simulink model "ARS308_RX"  (R2018b)
settings: Solver=FixedStepAuto  StartTime=0.0  StopTime=inf  FixedStep=0.005  RelTol=1e-3
PostLoadFcn:
  | if any(exist('dsrtsu_mdlpostloadfcn', 'file') ~= 0), dsrtsu_mdlpostloadfcn('Execute', bdroot); end
libraries: rtican x18
(part 3 of 4)

== system ARS308_RX/Subsystem/Function-Call Subsystem3 ==
  function : TriggerPort  TriggerType=function-call  VariantControl=Variant
  Cast To Single : DataTypeConversion  OutDataTypeStr=single
  Cast To Single1 : DataTypeConversion  OutDataTypeStr=single
  Cast To Single2 : DataTypeConversion  OutDataTypeStr=single
  Obj_0_Status : rtican/RTICAN Receive (RX)   Reserved1=[]  Reserved2=[]  Reserved3=[]  Reserved4=[]  SfcnMessage=[]  Msg_Struct=[]  BoardTypeNo=[]  BoardNo=[]  ChannelNo=[]  Parameters=[]  DialogFcn=[]  UnitName=[]  Revision=[]  UnitValues=[]  DSProperties=struct('RTI',struct('Version',uint32(5),'BlockType',struct('isSLSource',uint8(1),'isSLSink',uint8(1),'isHWSource',uint8(0),'isHWSink',uint8(0),'isSetup',uint8(0),'isInline',uint8(1),'isNonInline',uint8(0),'isInterrupt',uint8(0),'isChannelwise',uint8(0)),'IOBoardType','RTICAN','UnitType','MESSAGE','Identifier','RX','DialogType','MSVC','BlockSet','RTICAN','SlaveProcessor','CAN'))  RTIBlockInterface=struct('OutputPortsWidth',int32([1 1 1 1 1 1]),'OutputPortsActive',[1 1 1 1 1 1],'OutputPortsName',{{'Obj_InterfaceVersion','Obj_MeasCounter','Obj_NofObjects',['RX status'],['RX time'],['RX delta time']}},'OutputPortsDataType',{{'SS_DOUBLE','SS_DOUBLE','SS_DOUBLE','SS_DOUBLE','SS_DOUBLE','SS_DOUBLE'}},'OutputPortsLabel',{{'Obj_InterfaceVersion','Obj_MeasCounter','Obj_NofObjects','','',''}},'OutputPortsLabelMode','ON','InputPortsWidth',int32(0),'InputPortsActive',0,'DialogFcn','rtican_message_interface_gui','BlockDisplay',{{'','center'}},'IconTransparency','on','ParameterTunableNames',{{}},'InitLevel',3,'BlockName',struct('Token',{{'Obj_0_Status'}}),'SampleTime',{{-1}},'TriggerPort',{{'none'}},'EnablePort',{{'none'}})  RTIBlockParameters=struct('BoardTypeNo',{{1,'OFF',[]}},'BoardNo',{{3,'ON',[1 16]}},'ChannelNo',{{2,'ON',[1 2]}},'Parameters',{{struct('DataFileSupport',struct('DataFileSelectedMaster',1,'DataFileSelectedLocal',1,'DataFileName',['c:\users\石丽\desktop\zone\2020_demo\308\ars408_can_database_ch2 -new.dbc|c:\users\石丽\desktop\zone\2020_demo\308\ars408_can_database_ch0 -new.dbc|c:\users\石丽\desktop\zone\2020_demo\308\ars408_can_database_ch1-new.dbc|c:\users\石丽\desktop\zone\2020_demo\308\ars408_can_database_ch3-new.dbc|'],'DataFileDate',{{{['18-12月-2020 14:05:28']},{['18-12月-2020 14:05:27']},{['18-12月-2020 14:05:27']},{['18-12月-2020 14:05:26']}}},'SelectedFile','c:\users\石丽\desktop\zone\2020_demo\308\ars408_can_database_ch3-new.dbc'),'Options',struct('StatusSelected',1,'TimeSelected',1,'DeltaTimeSelected',1,'BytePortSelected',0,'MessageLengthSelected',0,'TriggerPort',struct('Selected',0,'TriggerType',0),'UserCoding',struct('Selected',0,'InterfaceFile','UserDecodingFile','FcnName','UserDecodeFcn','InportSelected',0,'InportWidth',1,'OutportSelected',0,'OutportWidth',1),'EnablePortSelected',0,'SignalOnPortnameSelected',1,'UseRXService',0),'Message',struct('MsgOnBlocknameSelected',1,'MsgName','Obj_0_Status','MsgIdFormat',0,'MsgId',1594,'MsgLength',4,'NumSignals',3,'SampleTime',-1,'Signal',struct('SgnName',{'Obj_InterfaceVersion','Obj_MeasCounter','Obj_NofObjects'},'SgnStartBit',{4,8,24},'SgnLength',{4,16,8},'SgnType',{0,0,0},'ModeValue',{-1,-1,-1},'DataType',{0,0,0},'ByteLayout',{2,2,2},'Factor',{1,1,1},'Offset',{0,0,0},'SgnComment',{{['Object CAN Interface Version Number']},{['Measurement Counter']},{['Number of Objects sent']}},'SgnUnit',{'','',''},'Min',{0,0,0},'Max',{16,65535,255},'SLDataType',{'SS_DOUBLE','SS_DOUBLE','SS_DOUBLE'}),'MsgIdNumFormat',1,'MsgComment',{{['Status information about object']}}),'Version',1.2,'general',struct('isFromLib',0)),'OFF',[]}},'GroupId',{{struct('Group',{{'RTICAN'}},'No',1,'Behavior',{{'NAMECHANGE'}},'BlockType',{{'SINK'}},'NameChangeFlag',0),'OFF',[]}},'SFcnRTICANMessage',{{struct('MsgType','RX','SFcnPortType','Scalar','MsgName','Obj_0_Status','MsgIdFormat','STD','MsgId',1594,'MsgLength',4,'NumSignals',3,'SampleTime',-1,'Signal',struct('SgnName',{'Obj_InterfaceVersion','Obj_MeasCounter','Obj_NofObjects'},'SgnStartBit',{4,8,24},'SgnLength',{4,16,8},'SgnType',{'standard','standard','standard'},'ModeValue',{-1,-1,-1},'DataType',{['unsigned int'],['unsigned int'],['unsigned int']},'ByteLayout',{['motorola back.'],['motorola back.'],['motorola back.']},'Factor',{1,1,1},'Offset',{0,0,0},'SLDataType',{'SS_DOUBLE','SS_DOUBLE','SS_DOUBLE'}),'StatusSelected','yes','TimeSelected','yes','DeltaTimeSelected','yes','BytePortSelected','no','MessageLengthSelected','no','TriggerPort',struct('Selected','no','TriggerType',0),'UserCoding',struct('Selected','no','InterfaceFile','UserDecodingFile','FcnName','UserDecodeFcn','InportSelected','no','InportWidth',1,'OutportSelected','no','OutportWidth',1),'EnablePortSelected','no','UseRXService','no','BoardType','DS1','BoardNo',3,'ControllerNo',2),'OFF',[]}},'TLCFileName',{{'rtican_rx_message','OFF',[]}})  RTISFcnParameters=struct('SFcnRTICANMessage','struct','TLCFileName','char')  RTIBlockParaDefault=struct('BoardTypeNo',4302,'BoardNo',1,'ChannelNo',1,'Parameters',struct('DataFileSupport',struct('DataFileSelectedMaster',0,'DataFileSelectedLocal',0,'DataFileName','','DataFileDate','','SelectedFile',['<no file selected>']),'Options',struct('StatusSelected',1,'TimeSelected',1,'DeltaTimeSelected',1,'BytePortSelected',0,'MessageLengthSelected',0,'TriggerPort',struct('Selected',0,'TriggerType','rising'),'UserCoding',struct('Selected',0,'InterfaceFile','UserDecodingFile','FcnName','UserDecodeFcn','InportSelected',0,'InportWidth',1,'OutportSelected',0,'OutportWidth',1),'EnablePortSelected',0,'SignalOnPortnameSelected',1,'UseRXService',0),'Message',struct('MsgOnBlocknameSelected',0,'MsgName',['RX Message'],'MsgIdFormat',0,'MsgId',100,'MsgLength',8,'NumSignals',1,'SampleTime',-1,'Signal',struct('SgnName',['RX signal'],'SgnStartBit',0,'SgnLength',8,'SgnType',0,'ModeValue',-1,'DataType',0,'SLDataType','SS_DOUBLE','ByteLayout',0,'Factor',1,'Offset',0,'Min',0,'Max',255,'SgnComment',{{}},'SgnUnit',''),'MsgIdNumFormat',0,'MsgComment',{{''}}),'Version',1.2,'general',struct('isFromLib',1)),'GroupId',struct('Group',{{'RTICAN'}},'No',1,'Behavior',{{'NAMECHANGE'}},'BlockType',{{'SINK'}},'NameChangeFlag',0),'SFcnRTICANMessage',struct('MsgType','RX','MsgName',['RX Message'],'MsgIdFormat','STD','MsgId',100,'MsgLength',8,'NumSignals',1,'SampleTime',-1,'Signal',struct('SgnName',['RX signal'],'SgnStartBit',0,'SgnLength',8,'SgnType','standard','ModeValue',-1,'DataType',['unsigned int'],'ByteLayout',['little endian'],'SLDataType','SS_DOUBLE','Factor',1,'Offset',0),'StatusSelected','yes','TimeSelected','yes','DeltaTimeSelected','yes','BytePortSelected','no','MessageLengthSelected','no','EnablePortSelected','no','UserCoding',struct('Selected','no','InterfaceFile','UserDecodingFile','FcnName','UserDecodeFcn','InportSelected','no','InportWidth',1,'OutportSelected','no','OutportWidth',1),'TriggerPort',struct('Selected','no','TriggerType','rising'),'UseRXService','no','BoardType','DS4302','BoardNo',1,'ControllerNo',1,'SFcnPortType','Scalar'),'TLCFileName','rtican_rx_message')
      settings: AttributesFormatString=Group Id: RTICAN1\n  SourceProductName=dSPACE RTI CAN Blockset
  Out1 : Outport
  Out2 : Outport  Port=2
  Out3 : Outport  Port=3
  wires:
  Obj_0_Status/2 -> Cast To Single/1  "Obj_MeasCounter"
  Obj_0_Status/3 -> Cast To Single1/1  "Obj_NofObjects"
  Cast To Single/1 -> Out1/1
  Cast To Single1/1 -> Out2/1
  Obj_0_Status/1 -> Cast To Single2/1  "Obj_InterfaceVersion"
  Cast To Single2/1 -> Out3/1

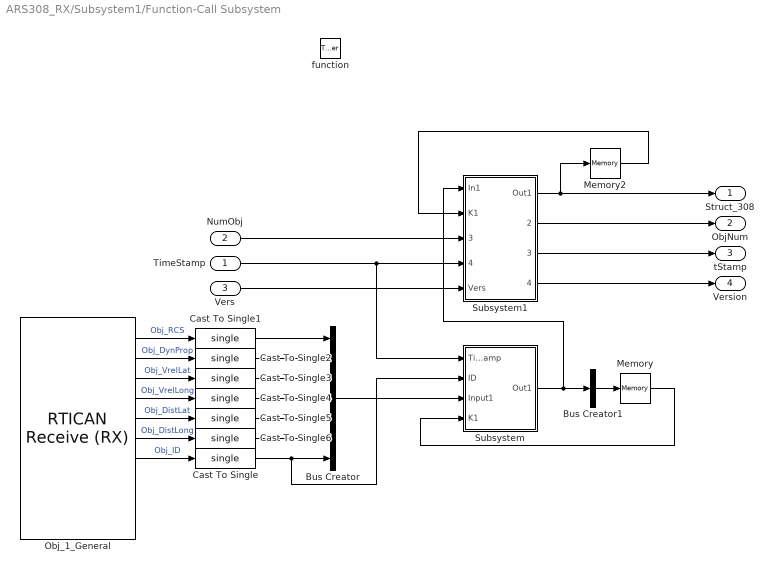
== system ARS308_RX/Subsystem1/Function-Call Subsystem ==
  TimeStamp : Inport
  NumObj : Inport  Port=2
  Vers : Inport  Port=3
  function : TriggerPort  TriggerType=function-call  VariantControl=Variant
  Bus Creator : BusCreator  Inputs=7  OutDataTypeStr=Bus: Bus_308  NonVirtualBus=on
      settings: InheritFromInputs=off
  Bus Creator1 : BusCreator  Inputs=1  OutDataTypeStr=Bus: BusArray_308  NonVirtualBus=on
      settings: InheritFromInputs=off
  Cast To Single{,1..6} (7 alike) : DataTypeConversion  OutDataTypeStr=single
  Memory : Memory  InheritSampleTime=on
  Memory2 : Memory  InheritSampleTime=on
  Obj_1_General : rtican/RTICAN Receive (RX)   Reserved1=[]  Reserved2=[]  Reserved3=[]  Reserved4=[]  SfcnMessage=[]  Msg_Struct=[]  BoardTypeNo=[]  BoardNo=[]  ChannelNo=[]  Parameters=[]  DialogFcn=[]  UnitName=[]  Revision=[]  UnitValues=[]  DSProperties=struct('RTI',struct('Version',uint32(5),'BlockType',struct('isSLSource',uint8(1),'isSLSink',uint8(1),'isHWSource',uint8(0),'isHWSink',uint8(0),'isSetup',uint8(0),'isInline',uint8(1),'isNonInline',uint8(0),'isInterrupt',uint8(0),'isChannelwise',uint8(0)),'IOBoardType','RTICAN','UnitType','MESSAGE','Identifier','RX','DialogType','MSVC','BlockSet','RTICAN','SlaveProcessor','CAN'))  RTIBlockInterface=struct('OutputPortsWidth',int32([1 1 1 1 1 1 1 1 1 1]),'OutputPortsActive',[1 1 1 1 1 1 1 1 1 1],'OutputPortsName',{{'Obj_RCS','Obj_DynProp','Obj_VrelLat','Obj_VrelLong','Obj_DistLat','Obj_DistLong','Obj_ID',['RX status'],['RX time'],['RX delta time']}},'OutputPortsDataType',{{'SS_DOUBLE','SS_DOUBLE','SS_DOUBLE','SS_DOUBLE','SS_DOUBLE','SS_DOUBLE','SS_DOUBLE','SS_DOUBLE','SS_DOUBLE','SS_DOUBLE'}},'OutputPortsLabel',{{'Obj_RCS','Obj_DynProp','Obj_VrelLat','Obj_VrelLong','Obj_DistLat','Obj_DistLong','Obj_ID','','',''}},'OutputPortsLabelMode','ON','InputPortsWidth',int32(0),'InputPortsActive',0,'DialogFcn','rtican_message_interface_gui','BlockDisplay',{{'','center'}},'IconTransparency','on','ParameterTunableNames',{{}},'InitLevel',3,'BlockName',struct('Token',{{'Obj_1_General'}}),'SampleTime',{{-1}},'TriggerPort',{{'none'}},'EnablePort',{{'none'}})  RTIBlockParameters=struct('BoardTypeNo',{{1,'OFF',[]}},'BoardNo',{{3,'ON',[1 16]}},'ChannelNo',{{1,'ON',[1 2]}},'Parameters',{{struct('DataFileSupport',struct('DataFileSelectedMaster',1,'DataFileSelectedLocal',1,'DataFileName',['c:\users\石丽\desktop\zone\2020_demo\308\ars408_can_database_ch0 -new.dbc|c:\users\石丽\desktop\zone\2020_demo\308\ars408_can_database_ch1-new.dbc|'],'DataFileDate',{{{['18-12月-2020 14:05:27']},{['18-12月-2020 14:05:27']}}},'SelectedFile',['c:\users\石丽\desktop\zone\2020_demo\308\ars408_can_database_ch0 -new.dbc']),'Options',struct('StatusSelected',1,'TimeSelected',1,'DeltaTimeSelected',1,'BytePortSelected',0,'MessageLengthSelected',0,'TriggerPort',struct('Selected',0,'TriggerType',0),'UserCoding',struct('Selected',0,'InterfaceFile','UserDecodingFile','FcnName','UserDecodeFcn','InportSelected',0,'InportWidth',1,'OutportSelected',0,'OutportWidth',1),'EnablePortSelected',0,'SignalOnPortnameSelected',1,'UseRXService',0),'Message',struct('MsgOnBlocknameSelected',1,'MsgName','Obj_1_General','MsgIdFormat',0,'MsgId',1547,'MsgLength',8,'NumSignals',7,'SampleTime',-1,'Signal',struct('SgnName',{'Obj_RCS','Obj_DynProp','Obj_VrelLat','Obj_VrelLong','Obj_DistLat','Obj_DistLong','Obj_ID'},'SgnStartBit',{0,8,13,22,32,43,56},'SgnLength',{8,3,9,10,11,13,8},'SgnType',{0,0,0,0,0,0,0},'ModeValue',{-1,-1,-1,-1,-1,-1,-1},'DataType',{0,0,0,0,0,0,0},'ByteLayout',{2,2,2,2,2,2,2},'Factor',{2^-1,1,2^-2,2^-2,0.2,0.2,1},'Offset',{-64,0,-64,-128,-204.6,-500,0},'SgnComment',{{['Object RCS value (radar cross section)']},{['Object dynamic property']},{['Object relative lateral velocity']},{['Object relative longitudinal velocity']},{['Object lateral displacement']},{['Object longitudinal displacement']},{['Object ID']}},'SgnUnit',{'dBm?','','m/s','m/s','m','m',''},'Min',{-64,0,-64,-128,-204.6,-500,0},'Max',{63.5,7,63.75,127.75,204.8,1138.2,255},'SLDataType',{'SS_DOUBLE','SS_DOUBLE','SS_DOUBLE','SS_DOUBLE','SS_DOUBLE','SS_DOUBLE','SS_DOUBLE'}),'MsgIdNumFormat',1,'MsgComment',{{['General object information']}}),'Version',1.2,'general',struct('isFromLib',0)),'OFF',[]}},'GroupId',{{struct('Group',{{'RTICAN'}},'No',2,'Behavior',{{'NAMECHANGE'}},'BlockType',{{'SINK'}},'NameChangeFlag',0),'OFF',[]}},'SFcnRTICANMessage',{{struct('MsgType','RX','SFcnPortType','Scalar','MsgName','Obj_1_General','MsgIdFormat','STD','MsgId',1547,'MsgLength',8,'NumSignals',7,'SampleTime',-1,'Signal',struct('SgnName',{'Obj_RCS','Obj_DynProp','Obj_VrelLat','Obj_VrelLong','Obj_DistLat','Obj_DistLong','Obj_ID'},'SgnStartBit',{0,8,13,22,32,43,56},'SgnLength',{8,3,9,10,11,13,8},'SgnType',{'standard','standard','standard','standard','standard','standard','standard'},'ModeValue',{-1,-1,-1,-1,-1,-1,-1},'DataType',{['unsigned int'],['unsigned int'],['unsigned int'],['unsigned int'],['unsigned int'],['unsigned int'],['unsigned int']},'ByteLayout',{['motorola back.'],['motorola back.'],['motorola back.'],['motorola back.'],['motorola back.'],['motorola back.'],['motorola back.']},'Factor',{2^-1,1,2^-2,2^-2,0.2,0.2,1},'Offset',{-64,0,-64,-128,-204.6,-500,0},'SLDataType',{'SS_DOUBLE','SS_DOUBLE','SS_DOUBLE','SS_DOUBLE','SS_DOUBLE','SS_DOUBLE','SS_DOUBLE'}),'StatusSelected','yes','TimeSelected','yes','DeltaTimeSelected','yes','BytePortSelected','no','MessageLengthSelected','no','TriggerPort',struct('Selected','no','TriggerType',0),'UserCoding',struct('Selected','no','InterfaceFile','UserDecodingFile','FcnName','UserDecodeFcn','InportSelected','no','InportWidth',1,'OutportSelected','no','OutportWidth',1),'EnablePortSelected','no','UseRXService','no','BoardType','DS1','BoardNo',3,'ControllerNo',1),'OFF',[]}},'TLCFileName',{{'rtican_rx_message','OFF',[]}})  RTISFcnParameters=struct('SFcnRTICANMessage','struct','TLCFileName','char')  RTIBlockParaDefault=struct('BoardTypeNo',4302,'BoardNo',1,'ChannelNo',1,'Parameters',struct('DataFileSupport',struct('DataFileSelectedMaster',0,'DataFileSelectedLocal',0,'DataFileName','','DataFileDate','','SelectedFile',['<no file selected>']),'Options',struct('StatusSelected',1,'TimeSelected',1,'DeltaTimeSelected',1,'BytePortSelected',0,'MessageLengthSelected',0,'TriggerPort',struct('Selected',0,'TriggerType','rising'),'UserCoding',struct('Selected',0,'InterfaceFile','UserDecodingFile','FcnName','UserDecodeFcn','InportSelected',0,'InportWidth',1,'OutportSelected',0,'OutportWidth',1),'EnablePortSelected',0,'SignalOnPortnameSelected',1,'UseRXService',0),'Message',struct('MsgOnBlocknameSelected',0,'MsgName',['RX Message'],'MsgIdFormat',0,'MsgId',100,'MsgLength',8,'NumSignals',1,'SampleTime',-1,'Signal',struct('SgnName',['RX signal'],'SgnStartBit',0,'SgnLength',8,'SgnType',0,'ModeValue',-1,'DataType',0,'SLDataType','SS_DOUBLE','ByteLayout',0,'Factor',1,'Offset',0,'Min',0,'Max',255,'SgnComment',{{}},'SgnUnit',''),'MsgIdNumFormat',0,'MsgComment',{{''}}),'Version',1.2,'general',struct('isFromLib',1)),'GroupId',struct('Group',{{'RTICAN'}},'No',1,'Behavior',{{'NAMECHANGE'}},'BlockType',{{'SINK'}},'NameChangeFlag',0),'SFcnRTICANMessage',struct('MsgType','RX','MsgName',['RX Message'],'MsgIdFormat','STD','MsgId',100,'MsgLength',8,'NumSignals',1,'SampleTime',-1,'Signal',struct('SgnName',['RX signal'],'SgnStartBit',0,'SgnLength',8,'SgnType','standard','ModeValue',-1,'DataType',['unsigned int'],'ByteLayout',['little endian'],'SLDataType','SS_DOUBLE','Factor',1,'Offset',0),'StatusSelected','yes','TimeSelected','yes','DeltaTimeSelected','yes','BytePortSelected','no','MessageLengthSelected','no','EnablePortSelected','no','UserCoding',struct('Selected','no','InterfaceFile','UserDecodingFile','FcnName','UserDecodeFcn','InportSelected','no','InportWidth',1,'OutportSelected','no','OutportWidth',1),'TriggerPort',struct('Selected','no','TriggerType','rising'),'UseRXService','no','BoardType','DS4302','BoardNo',1,'ControllerNo',1,'SFcnPortType','Scalar'),'TLCFileName','rtican_rx_message')
      settings: AttributesFormatString=Group Id: RTICAN2\n  SourceProductName=dSPACE RTI CAN Blockset
  Subsystem : Subsystem
  Subsystem1 : Subsystem
  Struct_308 : Outport  OutDataTypeStr=Bus: Bus_308
  ObjNum : Outport  Port=2
  tStamp : Outport  Port=3
  Version : Outport  Port=4
  wires:
  TimeStamp/1 -> Subsystem/1(TimeStamp), Subsystem1/4(TimeStamp)
  Subsystem/1(Out1) -> Bus Creator1/1, Subsystem1/1(In1)
  Cast To Single1/1 -> Bus Creator/1
  Bus Creator/1 -> Subsystem/3(Input1)
  Bus Creator1/1 -> Memory/1
  Memory/1 -> Subsystem/4(K1)
  NumObj/1 -> Subsystem1/3(NumObj)
  Subsystem1/1(Out1) -> Struct_308/1, Memory2/1
  Memory2/1 -> Subsystem1/2(K1)
  Subsystem1/2(ObjNum) -> ObjNum/1
  Subsystem1/3(tStamp) -> tStamp/1
  Cast To Single5/1 -> Bus Creator/5
  Cast To Single2/1 -> Bus Creator/2
  Cast To Single3/1 -> Bus Creator/3
  Cast To Single4/1 -> Bus Creator/4
  Cast To Single6/1 -> Bus Creator/6
  Cast To Single/1 -> Subsystem/2(ID), Bus Creator/7
  Vers/1 -> Subsystem1/5(Vers)
  Subsystem1/4(Version) -> Version/1
  Obj_1_General/1 -> Cast To Single1/1  "Obj_RCS"
  Obj_1_General/2 -> Cast To Single2/1  "Obj_DynProp"
  Obj_1_General/3 -> Cast To Single3/1  "Obj_VrelLat"
  Obj_1_General/4 -> Cast To Single4/1  "Obj_VrelLong"
  Obj_1_General/5 -> Cast To Single5/1  "Obj_DistLat"
  Obj_1_General/6 -> Cast To Single6/1  "Obj_DistLong"
  Obj_1_General/7 -> Cast To Single/1  "Obj_ID"

== system ARS308_RX/Subsystem1/Function-Call Subsystem1 ==
  function : TriggerPort  TriggerType=function-call  VariantControl=Variant
  Cast To Single : DataTypeConversion  OutDataTypeStr=single
  Cast To Single1 : DataTypeConversion  OutDataTypeStr=single
  Cast To Single2 : DataTypeConversion  OutDataTypeStr=single
  Obj_0_Status : rtican/RTICAN Receive (RX)   Reserved1=[]  Reserved2=[]  Reserved3=[]  Reserved4=[]  SfcnMessage=[]  Msg_Struct=[]  BoardTypeNo=[]  BoardNo=[]  ChannelNo=[]  Parameters=[]  DialogFcn=[]  UnitName=[]  Revision=[]  UnitValues=[]  DSProperties=struct('RTI',struct('Version',uint32(5),'BlockType',struct('isSLSource',uint8(1),'isSLSink',uint8(1),'isHWSource',uint8(0),'isHWSink',uint8(0),'isSetup',uint8(0),'isInline',uint8(1),'isNonInline',uint8(0),'isInterrupt',uint8(0),'isChannelwise',uint8(0)),'IOBoardType','RTICAN','UnitType','MESSAGE','Identifier','RX','DialogType','MSVC','BlockSet','RTICAN','SlaveProcessor','CAN'))  RTIBlockInterface=struct('OutputPortsWidth',int32([1 1 1 1 1 1]),'OutputPortsActive',[1 1 1 1 1 1],'OutputPortsName',{{'Obj_InterfaceVersion','Obj_MeasCounter','Obj_NofObjects',['RX status'],['RX time'],['RX delta time']}},'OutputPortsDataType',{{'SS_DOUBLE','SS_DOUBLE','SS_DOUBLE','SS_DOUBLE','SS_DOUBLE','SS_DOUBLE'}},'OutputPortsLabel',{{'Obj_InterfaceVersion','Obj_MeasCounter','Obj_NofObjects','','',''}},'OutputPortsLabelMode','ON','InputPortsWidth',int32(0),'InputPortsActive',0,'DialogFcn','rtican_message_interface_gui','BlockDisplay',{{'','center'}},'IconTransparency','on','ParameterTunableNames',{{}},'InitLevel',3,'BlockName',struct('Token',{{'Obj_0_Status'}}),'SampleTime',{{-1}},'TriggerPort',{{'none'}},'EnablePort',{{'none'}})  RTIBlockParameters=struct('BoardTypeNo',{{1,'OFF',[]}},'BoardNo',{{3,'ON',[1 16]}},'ChannelNo',{{1,'ON',[1 2]}},'Parameters',{{struct('DataFileSupport',struct('DataFileSelectedMaster',1,'DataFileSelectedLocal',1,'DataFileName',['c:\users\石丽\desktop\zone\2020_demo\308\ars408_can_database_ch0 -new.dbc|c:\users\石丽\desktop\zone\2020_demo\308\ars408_can_database_ch1-new.dbc|'],'DataFileDate',{{{['18-12月-2020 14:05:28']},{['18-12月-2020 14:05:26']}}},'SelectedFile',['c:\users\石丽\desktop\zone\2020_demo\308\ars408_can_database_ch0 -new.dbc']),'Options',struct('StatusSelected',1,'TimeSelected',1,'DeltaTimeSelected',1,'BytePortSelected',0,'MessageLengthSelected',0,'TriggerPort',struct('Selected',0,'TriggerType',0),'UserCoding',struct('Selected',0,'InterfaceFile','UserDecodingFile','FcnName','UserDecodeFcn','InportSelected',0,'InportWidth',1,'OutportSelected',0,'OutportWidth',1),'EnablePortSelected',0,'SignalOnPortnameSelected',1,'UseRXService',0),'Message',struct('MsgOnBlocknameSelected',1,'MsgName','Obj_0_Status','MsgIdFormat',0,'MsgId',1546,'MsgLength',4,'NumSignals',3,'SampleTime',-1,'Signal',struct('SgnName',{'Obj_InterfaceVersion','Obj_MeasCounter','Obj_NofObjects'},'SgnStartBit',{4,8,24},'SgnLength',{4,16,8},'SgnType',{0,0,0},'ModeValue',{-1,-1,-1},'DataType',{0,0,0},'ByteLayout',{2,2,2},'Factor',{1,1,1},'Offset',{0,0,0},'SgnComment',{{['Object CAN Interface Version Number']},{['Measurement Counter']},{['Number of Objects sent']}},'SgnUnit',{'','',''},'Min',{0,0,0},'Max',{16,65535,255},'SLDataType',{'SS_DOUBLE','SS_DOUBLE','SS_DOUBLE'}),'MsgIdNumFormat',1,'MsgComment',{{['Status information about object']}}),'Version',1.2,'general',struct('isFromLib',0)),'OFF',[]}},'GroupId',{{struct('Group',{{'RTICAN'}},'No',2,'Behavior',{{'NAMECHANGE'}},'BlockType',{{'SINK'}},'NameChangeFlag',0),'OFF',[]}},'SFcnRTICANMessage',{{struct('MsgType','RX','SFcnPortType','Scalar','MsgName','Obj_0_Status','MsgIdFormat','STD','MsgId',1546,'MsgLength',4,'NumSignals',3,'SampleTime',-1,'Signal',struct('SgnName',{'Obj_InterfaceVersion','Obj_MeasCounter','Obj_NofObjects'},'SgnStartBit',{4,8,24},'SgnLength',{4,16,8},'SgnType',{'standard','standard','standard'},'ModeValue',{-1,-1,-1},'DataType',{['unsigned int'],['unsigned int'],['unsigned int']},'ByteLayout',{['motorola back.'],['motorola back.'],['motorola back.']},'Factor',{1,1,1},'Offset',{0,0,0},'SLDataType',{'SS_DOUBLE','SS_DOUBLE','SS_DOUBLE'}),'StatusSelected','yes','TimeSelected','yes','DeltaTimeSelected','yes','BytePortSelected','no','MessageLengthSelected','no','TriggerPort',struct('Selected','no','TriggerType',0),'UserCoding',struct('Selected','no','InterfaceFile','UserDecodingFile','FcnName','UserDecodeFcn','InportSelected','no','InportWidth',1,'OutportSelected','no','OutportWidth',1),'EnablePortSelected','no','UseRXService','no','BoardType','DS1','BoardNo',3,'ControllerNo',2),'OFF',[]}},'TLCFileName',{{'rtican_rx_message','OFF',[]}})  RTISFcnParameters=struct('SFcnRTICANMessage','struct','TLCFileName','char')  RTIBlockParaDefault=struct('BoardTypeNo',4302,'BoardNo',1,'ChannelNo',1,'Parameters',struct('DataFileSupport',struct('DataFileSelectedMaster',0,'DataFileSelectedLocal',0,'DataFileName','','DataFileDate','','SelectedFile',['<no file selected>']),'Options',struct('StatusSelected',1,'TimeSelected',1,'DeltaTimeSelected',1,'BytePortSelected',0,'MessageLengthSelected',0,'TriggerPort',struct('Selected',0,'TriggerType','rising'),'UserCoding',struct('Selected',0,'InterfaceFile','UserDecodingFile','FcnName','UserDecodeFcn','InportSelected',0,'InportWidth',1,'OutportSelected',0,'OutportWidth',1),'EnablePortSelected',0,'SignalOnPortnameSelected',1,'UseRXService',0),'Message',struct('MsgOnBlocknameSelected',0,'MsgName',['RX Message'],'MsgIdFormat',0,'MsgId',100,'MsgLength',8,'NumSignals',1,'SampleTime',-1,'Signal',struct('SgnName',['RX signal'],'SgnStartBit',0,'SgnLength',8,'SgnType',0,'ModeValue',-1,'DataType',0,'SLDataType','SS_DOUBLE','ByteLayout',0,'Factor',1,'Offset',0,'Min',0,'Max',255,'SgnComment',{{}},'SgnUnit',''),'MsgIdNumFormat',0,'MsgComment',{{''}}),'Version',1.2,'general',struct('isFromLib',1)),'GroupId',struct('Group',{{'RTICAN'}},'No',1,'Behavior',{{'NAMECHANGE'}},'BlockType',{{'SINK'}},'NameChangeFlag',0),'SFcnRTICANMessage',struct('MsgType','RX','MsgName',['RX Message'],'MsgIdFormat','STD','MsgId',100,'MsgLength',8,'NumSignals',1,'SampleTime',-1,'Signal',struct('SgnName',['RX signal'],'SgnStartBit',0,'SgnLength',8,'SgnType','standard','ModeValue',-1,'DataType',['unsigned int'],'ByteLayout',['little endian'],'SLDataType','SS_DOUBLE','Factor',1,'Offset',0),'StatusSelected','yes','TimeSelected','yes','DeltaTimeSelected','yes','BytePortSelected','no','MessageLengthSelected','no','EnablePortSelected','no','UserCoding',struct('Selected','no','InterfaceFile','UserDecodingFile','FcnName','UserDecodeFcn','InportSelected','no','InportWidth',1,'OutportSelected','no','OutportWidth',1),'TriggerPort',struct('Selected','no','TriggerType','rising'),'UseRXService','no','BoardType','DS4302','BoardNo',1,'ControllerNo',1,'SFcnPortType','Scalar'),'TLCFileName','rtican_rx_message')
      settings: AttributesFormatString=Group Id: RTICAN2\n  SourceProductName=dSPACE RTI CAN Blockset
  Out1 : Outport
  Out2 : Outport  Port=2
  Out3 : Outport  Port=3
  wires:
  Obj_0_Status/2 -> Cast To Single/1  "Obj_MeasCounter"
  Obj_0_Status/3 -> Cast To Single1/1  "Obj_NofObjects"
  Cast To Single/1 -> Out1/1
  Cast To Single1/1 -> Out2/1
  Obj_0_Status/1 -> Cast To Single2/1  "Obj_InterfaceVersion"
  Cast To Single2/1 -> Out3/1

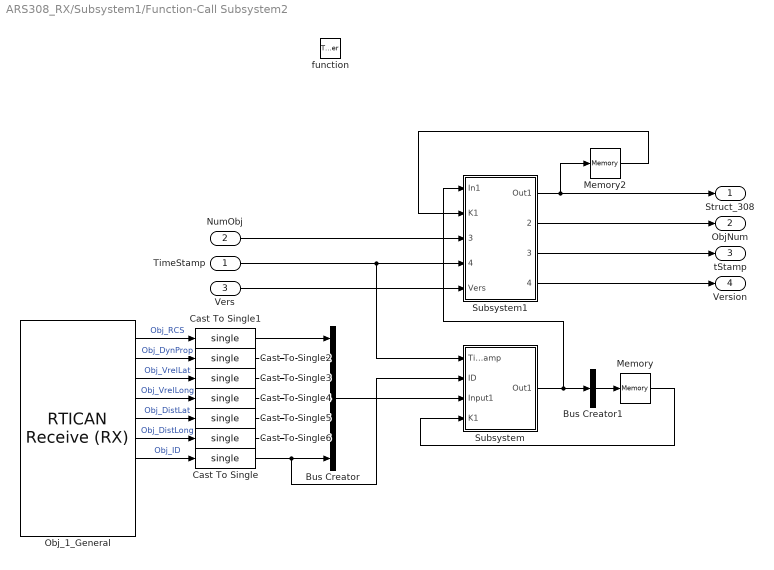
== system ARS308_RX/Subsystem1/Function-Call Subsystem2 ==
  TimeStamp : Inport
  NumObj : Inport  Port=2
  Vers : Inport  Port=3
  function : TriggerPort  TriggerType=function-call  VariantControl=Variant
  Bus Creator : BusCreator  Inputs=7  OutDataTypeStr=Bus: Bus_308  NonVirtualBus=on
      settings: InheritFromInputs=off
  Bus Creator1 : BusCreator  Inputs=1  OutDataTypeStr=Bus: BusArray_308  NonVirtualBus=on
      settings: InheritFromInputs=off
  Cast To Single{,1..6} (7 alike) : DataTypeConversion  OutDataTypeStr=single
  Memory : Memory  InheritSampleTime=on
  Memory2 : Memory  InheritSampleTime=on
  Obj_1_General : rtican/RTICAN Receive (RX)   Reserved1=[]  Reserved2=[]  Reserved3=[]  Reserved4=[]  SfcnMessage=[]  Msg_Struct=[]  BoardTypeNo=[]  BoardNo=[]  ChannelNo=[]  Parameters=[]  DialogFcn=[]  UnitName=[]  Revision=[]  UnitValues=[]  DSProperties=struct('RTI',struct('Version',uint32(5),'BlockType',struct('isSLSource',uint8(1),'isSLSink',uint8(1),'isHWSource',uint8(0),'isHWSink',uint8(0),'isSetup',uint8(0),'isInline',uint8(1),'isNonInline',uint8(0),'isInterrupt',uint8(0),'isChannelwise',uint8(0)),'IOBoardType','RTICAN','UnitType','MESSAGE','Identifier','RX','DialogType','MSVC','BlockSet','RTICAN','SlaveProcessor','CAN'))  RTIBlockInterface=struct('OutputPortsWidth',int32([1 1 1 1 1 1 1 1 1 1]),'OutputPortsActive',[1 1 1 1 1 1 1 1 1 1],'OutputPortsName',{{'Obj_RCS','Obj_DynProp','Obj_VrelLat','Obj_VrelLong','Obj_DistLat','Obj_DistLong','Obj_ID',['RX status'],['RX time'],['RX delta time']}},'OutputPortsDataType',{{'SS_DOUBLE','SS_DOUBLE','SS_DOUBLE','SS_DOUBLE','SS_DOUBLE','SS_DOUBLE','SS_DOUBLE','SS_DOUBLE','SS_DOUBLE','SS_DOUBLE'}},'OutputPortsLabel',{{'Obj_RCS','Obj_DynProp','Obj_VrelLat','Obj_VrelLong','Obj_DistLat','Obj_DistLong','Obj_ID','','',''}},'OutputPortsLabelMode','ON','InputPortsWidth',int32(0),'InputPortsActive',0,'DialogFcn','rtican_message_interface_gui','BlockDisplay',{{'','center'}},'IconTransparency','on','ParameterTunableNames',{{}},'InitLevel',3,'BlockName',struct('Token',{{'Obj_1_General'}}),'SampleTime',{{-1}},'TriggerPort',{{'none'}},'EnablePort',{{'none'}})  RTIBlockParameters=struct('BoardTypeNo',{{1,'OFF',[]}},'BoardNo',{{3,'ON',[1 16]}},'ChannelNo',{{1,'ON',[1 2]}},'Parameters',{{struct('DataFileSupport',struct('DataFileSelectedMaster',1,'DataFileSelectedLocal',1,'DataFileName',['c:\users\石丽\desktop\zone\2020_demo\308\ars408_can_database_ch0 -new.dbc|c:\users\石丽\desktop\zone\2020_demo\308\ars408_can_database_ch1-new.dbc|'],'DataFileDate',{{{['18-12月-2020 14:05:28']},{['18-12月-2020 14:05:26']}}},'SelectedFile','c:\users\石丽\desktop\zone\2020_demo\308\ars408_can_database_ch1-new.dbc'),'Options',struct('StatusSelected',1,'TimeSelected',1,'DeltaTimeSelected',1,'BytePortSelected',0,'MessageLengthSelected',0,'TriggerPort',struct('Selected',0,'TriggerType',0),'UserCoding',struct('Selected',0,'InterfaceFile','UserDecodingFile','FcnName','UserDecodeFcn','InportSelected',0,'InportWidth',1,'OutportSelected',0,'OutportWidth',1),'EnablePortSelected',0,'SignalOnPortnameSelected',1,'UseRXService',0),'Message',struct('MsgOnBlocknameSelected',1,'MsgName','Obj_1_General','MsgIdFormat',0,'MsgId',1563,'MsgLength',8,'NumSignals',7,'SampleTime',-1,'Signal',struct('SgnName',{'Obj_RCS','Obj_DynProp','Obj_VrelLat','Obj_VrelLong','Obj_DistLat','Obj_DistLong','Obj_ID'},'SgnStartBit',{0,8,13,22,32,43,56},'SgnLength',{8,3,9,10,11,13,8},'SgnType',{0,0,0,0,0,0,0},'ModeValue',{-1,-1,-1,-1,-1,-1,-1},'DataType',{0,0,0,0,0,0,0},'ByteLayout',{2,2,2,2,2,2,2},'Factor',{2^-1,1,2^-2,2^-2,0.2,0.2,1},'Offset',{-64,0,-64,-128,-204.6,-500,0},'SgnComment',{{['Object RCS value (radar cross section)']},{['Object dynamic property']},{['Object relative lateral velocity']},{['Object relative longitudinal velocity']},{['Object lateral displacement']},{['Object longitudinal displacement']},{['Object ID']}},'SgnUnit',{'dBm?','','m/s','m/s','m','m',''},'Min',{-64,0,-64,-128,-204.6,-500,0},'Max',{63.5,7,63.75,127.75,204.8,1138.2,255},'SLDataType',{'SS_DOUBLE','SS_DOUBLE','SS_DOUBLE','SS_DOUBLE','SS_DOUBLE','SS_DOUBLE','SS_DOUBLE'}),'MsgIdNumFormat',1,'MsgComment',{{['General object information']}}),'Version',1.2,'general',struct('isFromLib',0)),'OFF',[]}},'GroupId',{{struct('Group',{{'RTICAN'}},'No',2,'Behavior',{{'NAMECHANGE'}},'BlockType',{{'SINK'}},'NameChangeFlag',0),'OFF',[]}},'SFcnRTICANMessage',{{struct('MsgType','RX','SFcnPortType','Scalar','MsgName','Obj_1_General','MsgIdFormat','STD','MsgId',1563,'MsgLength',8,'NumSignals',7,'SampleTime',-1,'Signal',struct('SgnName',{'Obj_RCS','Obj_DynProp','Obj_VrelLat','Obj_VrelLong','Obj_DistLat','Obj_DistLong','Obj_ID'},'SgnStartBit',{0,8,13,22,32,43,56},'SgnLength',{8,3,9,10,11,13,8},'SgnType',{'standard','standard','standard','standard','standard','standard','standard'},'ModeValue',{-1,-1,-1,-1,-1,-1,-1},'DataType',{['unsigned int'],['unsigned int'],['unsigned int'],['unsigned int'],['unsigned int'],['unsigned int'],['unsigned int']},'ByteLayout',{['motorola back.'],['motorola back.'],['motorola back.'],['motorola back.'],['motorola back.'],['motorola back.'],['motorola back.']},'Factor',{2^-1,1,2^-2,2^-2,0.2,0.2,1},'Offset',{-64,0,-64,-128,-204.6,-500,0},'SLDataType',{'SS_DOUBLE','SS_DOUBLE','SS_DOUBLE','SS_DOUBLE','SS_DOUBLE','SS_DOUBLE','SS_DOUBLE'}),'StatusSelected','yes','TimeSelected','yes','DeltaTimeSelected','yes','BytePortSelected','no','MessageLengthSelected','no','TriggerPort',struct('Selected','no','TriggerType',0),'UserCoding',struct('Selected','no','InterfaceFile','UserDecodingFile','FcnName','UserDecodeFcn','InportSelected','no','InportWidth',1,'OutportSelected','no','OutportWidth',1),'EnablePortSelected','no','UseRXService','no','BoardType','DS1','BoardNo',3,'ControllerNo',1),'OFF',[]}},'TLCFileName',{{'rtican_rx_message','OFF',[]}})  RTISFcnParameters=struct('SFcnRTICANMessage','struct','TLCFileName','char')  RTIBlockParaDefault=struct('BoardTypeNo',4302,'BoardNo',1,'ChannelNo',1,'Parameters',struct('DataFileSupport',struct('DataFileSelectedMaster',0,'DataFileSelectedLocal',0,'DataFileName','','DataFileDate','','SelectedFile',['<no file selected>']),'Options',struct('StatusSelected',1,'TimeSelected',1,'DeltaTimeSelected',1,'BytePortSelected',0,'MessageLengthSelected',0,'TriggerPort',struct('Selected',0,'TriggerType','rising'),'UserCoding',struct('Selected',0,'InterfaceFile','UserDecodingFile','FcnName','UserDecodeFcn','InportSelected',0,'InportWidth',1,'OutportSelected',0,'OutportWidth',1),'EnablePortSelected',0,'SignalOnPortnameSelected',1,'UseRXService',0),'Message',struct('MsgOnBlocknameSelected',0,'MsgName',['RX Message'],'MsgIdFormat',0,'MsgId',100,'MsgLength',8,'NumSignals',1,'SampleTime',-1,'Signal',struct('SgnName',['RX signal'],'SgnStartBit',0,'SgnLength',8,'SgnType',0,'ModeValue',-1,'DataType',0,'SLDataType','SS_DOUBLE','ByteLayout',0,'Factor',1,'Offset',0,'Min',0,'Max',255,'SgnComment',{{}},'SgnUnit',''),'MsgIdNumFormat',0,'MsgComment',{{''}}),'Version',1.2,'general',struct('isFromLib',1)),'GroupId',struct('Group',{{'RTICAN'}},'No',1,'Behavior',{{'NAMECHANGE'}},'BlockType',{{'SINK'}},'NameChangeFlag',0),'SFcnRTICANMessage',struct('MsgType','RX','MsgName',['RX Message'],'MsgIdFormat','STD','MsgId',100,'MsgLength',8,'NumSignals',1,'SampleTime',-1,'Signal',struct('SgnName',['RX signal'],'SgnStartBit',0,'SgnLength',8,'SgnType','standard','ModeValue',-1,'DataType',['unsigned int'],'ByteLayout',['little endian'],'SLDataType','SS_DOUBLE','Factor',1,'Offset',0),'StatusSelected','yes','TimeSelected','yes','DeltaTimeSelected','yes','BytePortSelected','no','MessageLengthSelected','no','EnablePortSelected','no','UserCoding',struct('Selected','no','InterfaceFile','UserDecodingFile','FcnName','UserDecodeFcn','InportSelected','no','InportWidth',1,'OutportSelected','no','OutportWidth',1),'TriggerPort',struct('Selected','no','TriggerType','rising'),'UseRXService','no','BoardType','DS4302','BoardNo',1,'ControllerNo',1,'SFcnPortType','Scalar'),'TLCFileName','rtican_rx_message')
      settings: AttributesFormatString=Group Id: RTICAN2\n  SourceProductName=dSPACE RTI CAN Blockset
  Subsystem : Subsystem
  Subsystem1 : Subsystem
  Struct_308 : Outport  OutDataTypeStr=Bus: Bus_308
  ObjNum : Outport  Port=2
  tStamp : Outport  Port=3
  Version : Outport  Port=4
  wires:
  TimeStamp/1 -> Subsystem/1(TimeStamp), Subsystem1/4(TimeStamp)
  Subsystem/1(Out1) -> Bus Creator1/1, Subsystem1/1(In1)
  Obj_1_General/1 -> Cast To Single1/1  "Obj_RCS"
  Cast To Single1/1 -> Bus Creator/1
  Bus Creator/1 -> Subsystem/3(Input1)
  Bus Creator1/1 -> Memory/1
  Memory/1 -> Subsystem/4(K1)
  NumObj/1 -> Subsystem1/3(NumObj)
  Subsystem1/1(Out1) -> Struct_308/1, Memory2/1
  Memory2/1 -> Subsystem1/2(K1)
  Subsystem1/2(ObjNum) -> ObjNum/1
  Subsystem1/3(tStamp) -> tStamp/1
  Cast To Single5/1 -> Bus Creator/5
  Obj_1_General/6 -> Cast To Single6/1  "Obj_DistLong"
  Obj_1_General/5 -> Cast To Single5/1  "Obj_DistLat"
  Obj_1_General/4 -> Cast To Single4/1  "Obj_VrelLong"
  Obj_1_General/3 -> Cast To Single3/1  "Obj_VrelLat"
  Obj_1_General/2 -> Cast To Single2/1  "Obj_DynProp"
  Cast To Single2/1 -> Bus Creator/2
  Cast To Single3/1 -> Bus Creator/3
  Cast To Single4/1 -> Bus Creator/4
  Cast To Single6/1 -> Bus Creator/6
  Cast To Single/1 -> Subsystem/2(ID), Bus Creator/7
  Obj_1_General/7 -> Cast To Single/1  "Obj_ID"
  Vers/1 -> Subsystem1/5(Vers)
  Subsystem1/4(Version) -> Version/1

== system ARS308_RX/Subsystem1/Function-Call Subsystem3 ==
  function : TriggerPort  TriggerType=function-call  VariantControl=Variant
  Cast To Single : DataTypeConversion  OutDataTypeStr=single
  Cast To Single1 : DataTypeConversion  OutDataTypeStr=single
  Cast To Single2 : DataTypeConversion  OutDataTypeStr=single
  Obj_0_Status : rtican/RTICAN Receive (RX)   Reserved1=[]  Reserved2=[]  Reserved3=[]  Reserved4=[]  SfcnMessage=[]  Msg_Struct=[]  BoardTypeNo=[]  BoardNo=[]  ChannelNo=[]  Parameters=[]  DialogFcn=[]  UnitName=[]  Revision=[]  UnitValues=[]  DSProperties=struct('RTI',struct('Version',uint32(5),'BlockType',struct('isSLSource',uint8(1),'isSLSink',uint8(1),'isHWSource',uint8(0),'isHWSink',uint8(0),'isSetup',uint8(0),'isInline',uint8(1),'isNonInline',uint8(0),'isInterrupt',uint8(0),'isChannelwise',uint8(0)),'IOBoardType','RTICAN','UnitType','MESSAGE','Identifier','RX','DialogType','MSVC','BlockSet','RTICAN','SlaveProcessor','CAN'))  RTIBlockInterface=struct('OutputPortsWidth',int32([1 1 1 1 1 1]),'OutputPortsActive',[1 1 1 1 1 1],'OutputPortsName',{{'Obj_InterfaceVersion','Obj_MeasCounter','Obj_NofObjects',['RX status'],['RX time'],['RX delta time']}},'OutputPortsDataType',{{'SS_DOUBLE','SS_DOUBLE','SS_DOUBLE','SS_DOUBLE','SS_DOUBLE','SS_DOUBLE'}},'OutputPortsLabel',{{'Obj_InterfaceVersion','Obj_MeasCounter','Obj_NofObjects','','',''}},'OutputPortsLabelMode','ON','InputPortsWidth',int32(0),'InputPortsActive',0,'DialogFcn','rtican_message_interface_gui','BlockDisplay',{{'','center'}},'IconTransparency','on','ParameterTunableNames',{{}},'InitLevel',3,'BlockName',struct('Token',{{'Obj_0_Status'}}),'SampleTime',{{-1}},'TriggerPort',{{'none'}},'EnablePort',{{'none'}})  RTIBlockParameters=struct('BoardTypeNo',{{1,'OFF',[]}},'BoardNo',{{3,'ON',[1 16]}},'ChannelNo',{{1,'ON',[1 2]}},'Parameters',{{struct('DataFileSupport',struct('DataFileSelectedMaster',1,'DataFileSelectedLocal',1,'DataFileName',['c:\users\石丽\desktop\zone\2020_demo\308\ars408_can_database_ch0 -new.dbc|c:\users\石丽\desktop\zone\2020_demo\308\ars408_can_database_ch1-new.dbc|'],'DataFileDate',{{{['18-12月-2020 14:05:28']},{['18-12月-2020 14:05:26']}}},'SelectedFile','c:\users\石丽\desktop\zone\2020_demo\308\ars408_can_database_ch1-new.dbc'),'Options',struct('StatusSelected',1,'TimeSelected',1,'DeltaTimeSelected',1,'BytePortSelected',0,'MessageLengthSelected',0,'TriggerPort',struct('Selected',0,'TriggerType',0),'UserCoding',struct('Selected',0,'InterfaceFile','UserDecodingFile','FcnName','UserDecodeFcn','InportSelected',0,'InportWidth',1,'OutportSelected',0,'OutportWidth',1),'EnablePortSelected',0,'SignalOnPortnameSelected',1,'UseRXService',0),'Message',struct('MsgOnBlocknameSelected',1,'MsgName','Obj_0_Status','MsgIdFormat',0,'MsgId',1562,'MsgLength',4,'NumSignals',3,'SampleTime',-1,'Signal',struct('SgnName',{'Obj_InterfaceVersion','Obj_MeasCounter','Obj_NofObjects'},'SgnStartBit',{4,8,24},'SgnLength',{4,16,8},'SgnType',{0,0,0},'ModeValue',{-1,-1,-1},'DataType',{0,0,0},'ByteLayout',{2,2,2},'Factor',{1,1,1},'Offset',{0,0,0},'SgnComment',{{['Object CAN Interface Version Number']},{['Measurement Counter']},{['Number of Objects sent']}},'SgnUnit',{'','',''},'Min',{0,0,0},'Max',{16,65535,255},'SLDataType',{'SS_DOUBLE','SS_DOUBLE','SS_DOUBLE'}),'MsgIdNumFormat',1,'MsgComment',{{['Status information about object']}}),'Version',1.2,'general',struct('isFromLib',0)),'OFF',[]}},'GroupId',{{struct('Group',{{'RTICAN'}},'No',2,'Behavior',{{'NAMECHANGE'}},'BlockType',{{'SINK'}},'NameChangeFlag',0),'OFF',[]}},'SFcnRTICANMessage',{{struct('MsgType','RX','SFcnPortType','Scalar','MsgName','Obj_0_Status','MsgIdFormat','STD','MsgId',1562,'MsgLength',4,'NumSignals',3,'SampleTime',-1,'Signal',struct('SgnName',{'Obj_InterfaceVersion','Obj_MeasCounter','Obj_NofObjects'},'SgnStartBit',{4,8,24},'SgnLength',{4,16,8},'SgnType',{'standard','standard','standard'},'ModeValue',{-1,-1,-1},'DataType',{['unsigned int'],['unsigned int'],['unsigned int']},'ByteLayout',{['motorola back.'],['motorola back.'],['motorola back.']},'Factor',{1,1,1},'Offset',{0,0,0},'SLDataType',{'SS_DOUBLE','SS_DOUBLE','SS_DOUBLE'}),'StatusSelected','yes','TimeSelected','yes','DeltaTimeSelected','yes','BytePortSelected','no','MessageLengthSelected','no','TriggerPort',struct('Selected','no','TriggerType',0),'UserCoding',struct('Selected','no','InterfaceFile','UserDecodingFile','FcnName','UserDecodeFcn','InportSelected','no','InportWidth',1,'OutportSelected','no','OutportWidth',1),'EnablePortSelected','no','UseRXService','no','BoardType','DS1','BoardNo',3,'ControllerNo',1),'OFF',[]}},'TLCFileName',{{'rtican_rx_message','OFF',[]}})  RTISFcnParameters=struct('SFcnRTICANMessage','struct','TLCFileName','char')  RTIBlockParaDefault=struct('BoardTypeNo',4302,'BoardNo',1,'ChannelNo',1,'Parameters',struct('DataFileSupport',struct('DataFileSelectedMaster',0,'DataFileSelectedLocal',0,'DataFileName','','DataFileDate','','SelectedFile',['<no file selected>']),'Options',struct('StatusSelected',1,'TimeSelected',1,'DeltaTimeSelected',1,'BytePortSelected',0,'MessageLengthSelected',0,'TriggerPort',struct('Selected',0,'TriggerType','rising'),'UserCoding',struct('Selected',0,'InterfaceFile','UserDecodingFile','FcnName','UserDecodeFcn','InportSelected',0,'InportWidth',1,'OutportSelected',0,'OutportWidth',1),'EnablePortSelected',0,'SignalOnPortnameSelected',1,'UseRXService',0),'Message',struct('MsgOnBlocknameSelected',0,'MsgName',['RX Message'],'MsgIdFormat',0,'MsgId',100,'MsgLength',8,'NumSignals',1,'SampleTime',-1,'Signal',struct('SgnName',['RX signal'],'SgnStartBit',0,'SgnLength',8,'SgnType',0,'ModeValue',-1,'DataType',0,'SLDataType','SS_DOUBLE','ByteLayout',0,'Factor',1,'Offset',0,'Min',0,'Max',255,'SgnComment',{{}},'SgnUnit',''),'MsgIdNumFormat',0,'MsgComment',{{''}}),'Version',1.2,'general',struct('isFromLib',1)),'GroupId',struct('Group',{{'RTICAN'}},'No',1,'Behavior',{{'NAMECHANGE'}},'BlockType',{{'SINK'}},'NameChangeFlag',0),'SFcnRTICANMessage',struct('MsgType','RX','MsgName',['RX Message'],'MsgIdFormat','STD','MsgId',100,'MsgLength',8,'NumSignals',1,'SampleTime',-1,'Signal',struct('SgnName',['RX signal'],'SgnStartBit',0,'SgnLength',8,'SgnType','standard','ModeValue',-1,'DataType',['unsigned int'],'ByteLayout',['little endian'],'SLDataType','SS_DOUBLE','Factor',1,'Offset',0),'StatusSelected','yes','TimeSelected','yes','DeltaTimeSelected','yes','BytePortSelected','no','MessageLengthSelected','no','EnablePortSelected','no','UserCoding',struct('Selected','no','InterfaceFile','UserDecodingFile','FcnName','UserDecodeFcn','InportSelected','no','InportWidth',1,'OutportSelected','no','OutportWidth',1),'TriggerPort',struct('Selected','no','TriggerType','rising'),'UseRXService','no','BoardType','DS4302','BoardNo',1,'ControllerNo',1,'SFcnPortType','Scalar'),'TLCFileName','rtican_rx_message')
      settings: AttributesFormatString=Group Id: RTICAN2\n  SourceProductName=dSPACE RTI CAN Blockset
  Out1 : Outport
  Out2 : Outport  Port=2
  Out3 : Outport  Port=3
  wires:
  Obj_0_Status/2 -> Cast To Single/1  "Obj_MeasCounter"
  Obj_0_Status/3 -> Cast To Single1/1  "Obj_NofObjects"
  Cast To Single/1 -> Out1/1
  Cast To Single1/1 -> Out2/1
  Obj_0_Status/1 -> Cast To Single2/1  "Obj_InterfaceVersion"
  Cast To Single2/1 -> Out3/1

== system ARS308_RX/RTI Data/RTI Data Store/RTI Data Store ==
  RTI Data Store : Subsystem  mask(RTI_DATA_STORE){}
      mask help:
      | RTI Data Store Block. This block is used by RTI to store internal model dependent data. Deleting this block will result in data loss.
      |
      | NEVER DELETE, COPY, OR MODIFY THIS BLOCK!
      mask Help:
      | RTI Data Store Block. This block is used by RTI to store internal model dependent data. Deleting this block will result in data loss.
      | 
      | NEVER DELETE, COPY, OR MODIFY THIS BLOCK!
      mask Display: text(0.5, 0.5, ' ', 'HorizontalAlignment', 'center');

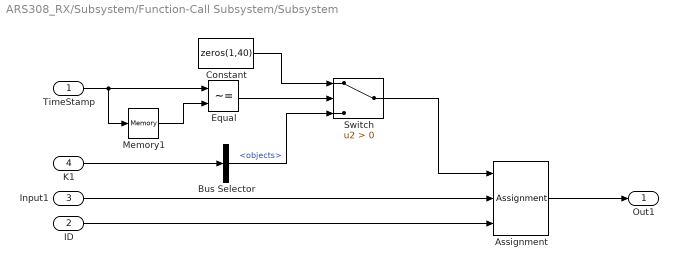
== system ARS308_RX/Subsystem/Function-Call Subsystem/Subsystem ==
  TimeStamp : Inport
  ID : Inport  Port=2
  Input1 : Inport  Port=3
  K1 : Inport  Port=4  OutDataTypeStr=Bus: BusArray_308
  Assignment : Assignment  IndexMode=Zero-based  DiagnosticForDimensions=Warning  IndexOptions=Index vector (port)  Indices=1  OutputSizes=1
  Bus Selector : BusSelector  OutputSignals=objects
  Constant : Constant  Value=zeros(1,40)  OutDataTypeStr=Bus: Bus_308
  Equal : RelationalOperator  Operator=~=  OutDataTypeStr=boolean  RndMeth=Simplest
  Memory1 : Memory  InheritSampleTime=on
  Switch : Switch  Criteria=u2 > Threshold
  Out1 : Outport  OutDataTypeStr=Bus: Bus_308
  wires:
  TimeStamp/1 -> Memory1/1, Equal/1
  Memory1/1 -> Equal/2
  Constant/1 -> Switch/1
  Equal/1 -> Switch/2
  Input1/1 -> Assignment/2
  ID/1 -> Assignment/3
  K1/1 -> Bus Selector/1
  Bus Selector/1 -> Switch/3  "<objects>"
  Switch/1 -> Assignment/1
  Assignment/1 -> Out1/1

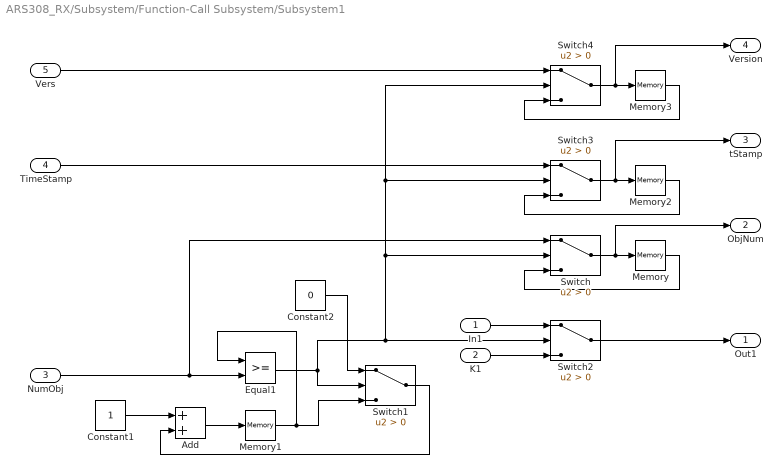
== system ARS308_RX/Subsystem/Function-Call Subsystem/Subsystem1 ==
  In1 : Inport
  K1 : Inport  Port=2
  NumObj : Inport  Port=3
  TimeStamp : Inport  Port=4
  Vers : Inport  Port=5
  Add : Sum
  Constant1 : Constant  OutDataTypeStr=single
  Constant2 : Constant  Value=0  OutDataTypeStr=single
  Equal1 : RelationalOperator  OutDataTypeStr=boolean  RndMeth=Simplest
  Memory : Memory  InheritSampleTime=on
  Memory1 : Memory  InitialCondition=1  InheritSampleTime=on
  Memory2 : Memory  InheritSampleTime=on
  Memory3 : Memory  InheritSampleTime=on
  Switch{,1..4} (5 alike) : Switch  Criteria=u2 > Threshold
  Out1 : Outport
  ObjNum : Outport  Port=2
  tStamp : Outport  Port=3
  Version : Outport  Port=4
  wires:
  Constant1/1 -> Add/1
  NumObj/1 -> Switch/1, Equal1/2
  K1/1 -> Switch2/3
  Constant2/1 -> Switch1/1
  Switch2/1 -> Out1/1
  Add/1 -> Memory1/1
  In1/1 -> Switch2/1
  Switch/1 -> ObjNum/1, Memory/1
  Memory/1 -> Switch/3
  Memory1/1 -> Equal1/1, Switch1/3
  Switch1/1 -> Add/2
  TimeStamp/1 -> Switch3/1
  Switch3/1 -> tStamp/1, Memory2/1
  Memory2/1 -> Switch3/3
  Equal1/1 -> Switch4/2, Switch3/2, Switch/2, Switch2/2, Switch1/2
  Memory3/1 -> Switch4/3
  Switch4/1 -> Version/1, Memory3/1
  Vers/1 -> Switch4/1

== system ARS308_RX/Subsystem/Function-Call Subsystem2/Subsystem ==
  TimeStamp : Inport
  ID : Inport  Port=2
  Input1 : Inport  Port=3
  K1 : Inport  Port=4  OutDataTypeStr=Bus: BusArray_308
  Assignment : Assignment  IndexMode=Zero-based  DiagnosticForDimensions=Warning  IndexOptions=Index vector (port)  Indices=1  OutputSizes=1
  Bus Selector : BusSelector  OutputSignals=objects
  Constant : Constant  Value=zeros(1,40)  OutDataTypeStr=Bus: Bus_308
  Equal : RelationalOperator  Operator=~=  OutDataTypeStr=boolean  RndMeth=Simplest
  Memory1 : Memory  InheritSampleTime=on
  Switch : Switch  Criteria=u2 > Threshold
  Out1 : Outport  OutDataTypeStr=Bus: Bus_308
  wires:
  TimeStamp/1 -> Memory1/1, Equal/1
  Memory1/1 -> Equal/2
  Constant/1 -> Switch/1
  Equal/1 -> Switch/2
  Input1/1 -> Assignment/2
  ID/1 -> Assignment/3
  K1/1 -> Bus Selector/1
  Bus Selector/1 -> Switch/3  "<objects>"
  Switch/1 -> Assignment/1
  Assignment/1 -> Out1/1

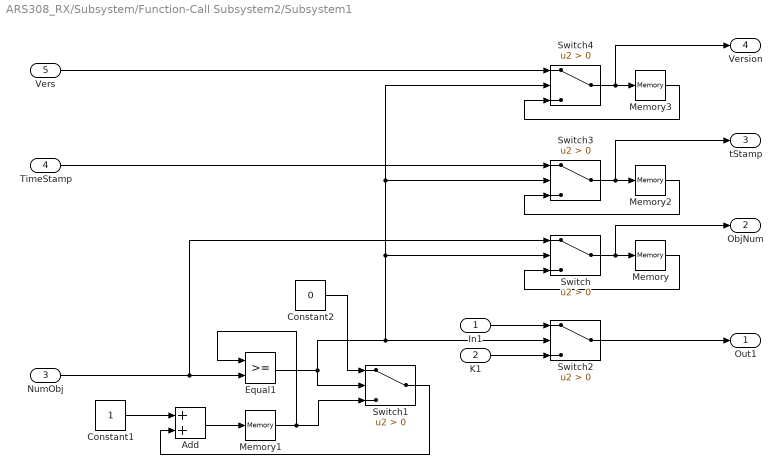
== system ARS308_RX/Subsystem/Function-Call Subsystem2/Subsystem1 ==
  In1 : Inport
  K1 : Inport  Port=2
  NumObj : Inport  Port=3
  TimeStamp : Inport  Port=4
  Vers : Inport  Port=5
  Add : Sum
  Constant1 : Constant  OutDataTypeStr=single
  Constant2 : Constant  Value=0  OutDataTypeStr=single
  Equal1 : RelationalOperator  OutDataTypeStr=boolean  RndMeth=Simplest
  Memory : Memory  InheritSampleTime=on
  Memory1 : Memory  InitialCondition=1  InheritSampleTime=on
  Memory2 : Memory  InheritSampleTime=on
  Memory3 : Memory  InheritSampleTime=on
  Switch{,1..4} (5 alike) : Switch  Criteria=u2 > Threshold
  Out1 : Outport
  ObjNum : Outport  Port=2
  tStamp : Outport  Port=3
  Version : Outport  Port=4
  wires:
  Constant1/1 -> Add/1
  NumObj/1 -> Switch/1, Equal1/2
  K1/1 -> Switch2/3
  Constant2/1 -> Switch1/1
  Switch2/1 -> Out1/1
  Add/1 -> Memory1/1
  In1/1 -> Switch2/1
  Switch/1 -> ObjNum/1, Memory/1
  Memory/1 -> Switch/3
  Memory1/1 -> Equal1/1, Switch1/3
  Switch1/1 -> Add/2
  TimeStamp/1 -> Switch3/1
  Switch3/1 -> tStamp/1, Memory2/1
  Memory2/1 -> Switch3/3
  Equal1/1 -> Switch4/2, Switch3/2, Switch/2, Switch2/2, Switch1/2
  Memory3/1 -> Switch4/3
  Switch4/1 -> Version/1, Memory3/1
  Vers/1 -> Switch4/1

== system ARS308_RX/Subsystem1/Function-Call Subsystem/Subsystem ==
  TimeStamp : Inport
  ID : Inport  Port=2
  Input1 : Inport  Port=3
  K1 : Inport  Port=4  OutDataTypeStr=Bus: BusArray_308
  Assignment : Assignment  IndexMode=Zero-based  DiagnosticForDimensions=Warning  IndexOptions=Index vector (port)  Indices=1  OutputSizes=1
  Bus Selector : BusSelector  OutputSignals=objects
  Constant : Constant  Value=zeros(1,40)  OutDataTypeStr=Bus: Bus_308
  Equal : RelationalOperator  Operator=~=  OutDataTypeStr=boolean  RndMeth=Simplest
  Memory1 : Memory  InheritSampleTime=on
  Switch : Switch  Criteria=u2 > Threshold
  Out1 : Outport  OutDataTypeStr=Bus: Bus_308
  wires:
  TimeStamp/1 -> Memory1/1, Equal/1
  Memory1/1 -> Equal/2
  Constant/1 -> Switch/1
  Equal/1 -> Switch/2
  Input1/1 -> Assignment/2
  ID/1 -> Assignment/3
  K1/1 -> Bus Selector/1
  Bus Selector/1 -> Switch/3  "<objects>"
  Switch/1 -> Assignment/1
  Assignment/1 -> Out1/1

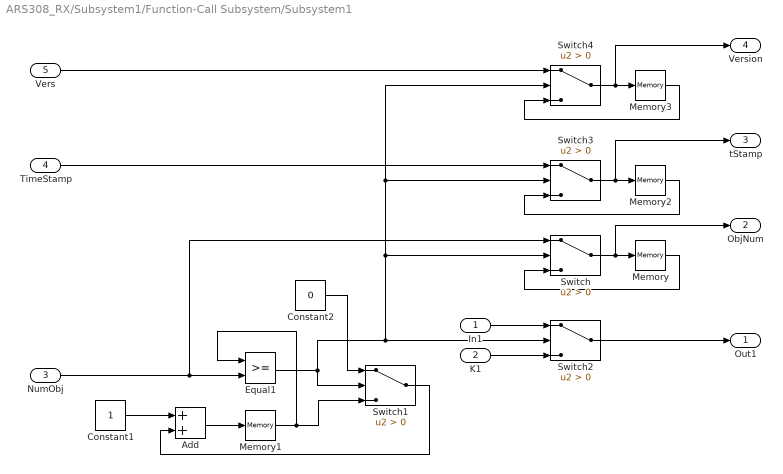
== system ARS308_RX/Subsystem1/Function-Call Subsystem/Subsystem1 ==
  In1 : Inport
  K1 : Inport  Port=2
  NumObj : Inport  Port=3
  TimeStamp : Inport  Port=4
  Vers : Inport  Port=5
  Add : Sum
  Constant1 : Constant  OutDataTypeStr=single
  Constant2 : Constant  Value=0  OutDataTypeStr=single
  Equal1 : RelationalOperator  OutDataTypeStr=boolean  RndMeth=Simplest
  Memory : Memory  InheritSampleTime=on
  Memory1 : Memory  InitialCondition=1  InheritSampleTime=on
  Memory2 : Memory  InheritSampleTime=on
  Memory3 : Memory  InheritSampleTime=on
  Switch{,1..4} (5 alike) : Switch  Criteria=u2 > Threshold
  Out1 : Outport
  ObjNum : Outport  Port=2
  tStamp : Outport  Port=3
  Version : Outport  Port=4
  wires:
  Constant1/1 -> Add/1
  NumObj/1 -> Switch/1, Equal1/2
  K1/1 -> Switch2/3
  Constant2/1 -> Switch1/1
  Switch2/1 -> Out1/1
  Add/1 -> Memory1/1
  In1/1 -> Switch2/1
  Switch/1 -> ObjNum/1, Memory/1
  Memory/1 -> Switch/3
  Memory1/1 -> Equal1/1, Switch1/3
  Switch1/1 -> Add/2
  TimeStamp/1 -> Switch3/1
  Switch3/1 -> tStamp/1, Memory2/1
  Memory2/1 -> Switch3/3
  Equal1/1 -> Switch4/2, Switch3/2, Switch/2, Switch2/2, Switch1/2
  Memory3/1 -> Switch4/3
  Switch4/1 -> Version/1, Memory3/1
  Vers/1 -> Switch4/1

== system ARS308_RX/Subsystem1/Function-Call Subsystem2/Subsystem ==
  TimeStamp : Inport
  ID : Inport  Port=2
  Input1 : Inport  Port=3
  K1 : Inport  Port=4  OutDataTypeStr=Bus: BusArray_308
  Assignment : Assignment  IndexMode=Zero-based  DiagnosticForDimensions=Warning  IndexOptions=Index vector (port)  Indices=1  OutputSizes=1
  Bus Selector : BusSelector  OutputSignals=objects
  Constant : Constant  Value=zeros(1,40)  OutDataTypeStr=Bus: Bus_308
  Equal : RelationalOperator  Operator=~=  OutDataTypeStr=boolean  RndMeth=Simplest
  Memory1 : Memory  InheritSampleTime=on
  Switch : Switch  Criteria=u2 > Threshold
  Out1 : Outport  OutDataTypeStr=Bus: Bus_308
  wires:
  TimeStamp/1 -> Memory1/1, Equal/1
  Memory1/1 -> Equal/2
  Constant/1 -> Switch/1
  Equal/1 -> Switch/2
  Input1/1 -> Assignment/2
  ID/1 -> Assignment/3
  K1/1 -> Bus Selector/1
  Bus Selector/1 -> Switch/3  "<objects>"
  Switch/1 -> Assignment/1
  Assignment/1 -> Out1/1
